simulink model "carmen_controller_HOST_prev"  (R2013b)
settings: Solver=FixedStepDiscrete  StartTime=0.0  StopTime=inf  FixedStep=0.01  RelTol=1e-3
PreLoadFcn:
  | load('motor_rule.mat');
values from neighbouring files (symbols this model uses):
  amplitud = 27000    [setup.m]
  frec = 0.1    [setup.m]
libraries: simulink x2
settings Model: Creator=Sr Antonio  LastModifiedBy=Cristina
settings DataIOCC: SignalLoggingSaveFormat=ModelDataLogs
settings OptimizationCC: ExpressionDepthLimit=2147483647
settings DebuggingCC: FcnCallInpInsideContextMsg=EnableAllAsWarning  StateNameClashWarn=warning
settings GRTTargetCC: CombineOutputUpdateFcns=off  GRTInterface=on

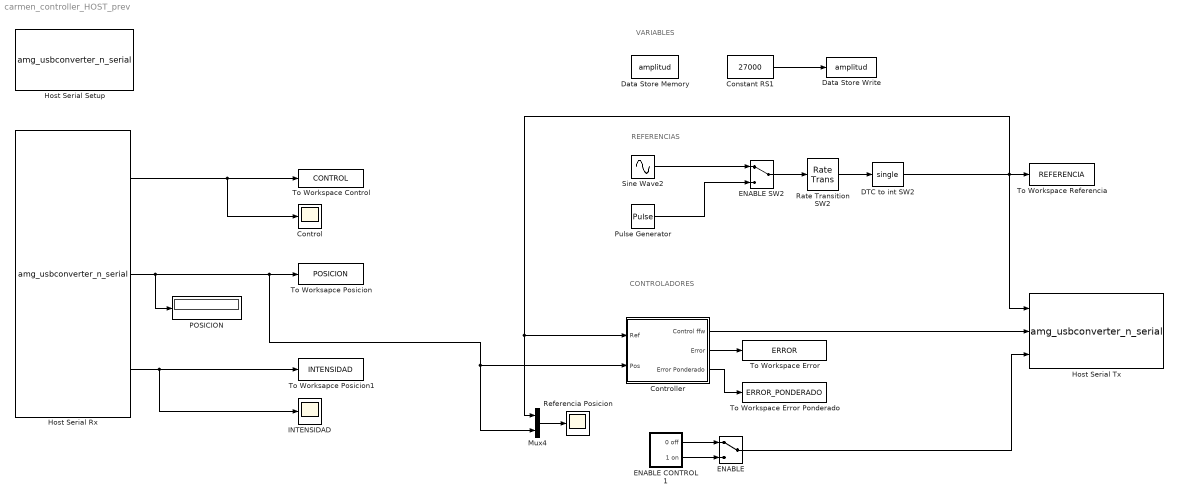
== system carmen_controller_HOST_prev ==
  note: REFERENCIAS
  note: CONTROLADORES
  note: VARIABLES
  Constant RS1 : Constant  Value=27000  OutDataTypeStr=single  SampleTime=0.01
  Control : Scope
      settings: TimeRange=10  YMin=0  YMax=37.5
  Controller : Subsystem
  DTC to int SW2 : DataTypeConversion  OutDataTypeStr=single
  Data Store Memory : DataStoreMemory  DataStoreName=amplitud  ReadBeforeWriteMsg=warning  WriteAfterWriteMsg=warning  WriteAfterReadMsg=warning
  Data Store Write : DataStoreWrite  DataStoreName=amplitud
  ENABLE : ManualSwitch
  ENABLE SW2 : ManualSwitch
  ENABLE CONTROL 1 : Subsystem
  Host Serial Rx : S-Function  Priority=1  FunctionName=amg_usbconverter_n_serial  Parameters=configuration,port,transfer,baudrate,stopbit,inputtype,outputtype,binheaderarray,binterminatorarray,asciiheader,asciiterminator,bindatalength,packetmode,timeout,sampletime,initialvalues,blockid  EnableBusSupport=off  mask(amg_usbconverter_n_serial){configuration=Rx, port=COM3, baudrate=115200, databits=8, parity=None, stopbit=1, flowcontrol=None, advanceoptions=off, rxbuffersize=2048, txbuffersize=2048, transfer=Blocking, enableinitial=off, initialvalues=[], timeout=2, packetmode=Binary, binheader='0E 0E', binterminator='0A 0A', porttype_double=0, porttype_single=3, porttype_int8=0, porttype_uint8=0, porttype_int16=0, porttype_uint16=0, porttype_int32=0, porttype_uint32=0, asciiformat='%d,%f', rx_asciiterminator=LF (0x0A - "\n"), tx_asciiterminator=LF (0x0A - "\n"), inputtype=[0], outputtype=[3  1 1 1], binheaderarray=[2 14  14], binterminatorarray=[2 10  10], bindatalength=12, asciiheader=['%d,%f' uint8(10)], asciiterminator=[1 10], sampletime=0.01, sampletimestr=, blockid=HostSerialRx}
      mask prompts: baudrate "Baud rate (bps)"; databits "Data bits"; stopbit "Stop bit"; flowcontrol "Hardware flow control"; advanceoptions "Advance options"; rxbuffersize "Rx buffer size (bytes)"; txbuffersize "Tx buffer size (bytes)"; enableinitial "Enable initial value  (Closed loop HIL test)"; initialvalues "Initial values"; timeout "Wait time-out (Seconds)"; packetmode "Packet mode"; binheader "Binary header (example: '7E 7E')"; binterminator "Binary terminator (example: '03 03')"; porttype_double "Number of data port, type DOUBLE"; porttype_single "Number of data port, type SINGLE"; porttype_int8 "Number of data port, type INT8"; porttype_uint8 "Number of data port, type UINT8"; porttype_int16 "Number of data port, type INT16"; porttype_uint16 "Number of data port, type UINT16"; porttype_int32 "Number of data port, type INT32"; porttype_uint32 "Number of data port, type UINT32"; asciiformat "Ascii format"; rx_asciiterminator "End of packet"; tx_asciiterminator "End of packet"; inputtype "Input data type"; outputtype "Output data type"; binheaderarray "Binary header"; binterminatorarray "Binary terminator"; bindatalength "Binary data length"; asciiheader "Ascii header (printf format)"; asciiterminator "Ascii terminator"; sampletime "Sample time (sec)"; sampletimestr "Compiled sample time (sec) in string"
      mask help:
      | Enable initial value (Closed loop HIL test):
      |  - Checked: The block will return a initial value (constant) at first time step.
      |  - Unchecked: Normal operation, the block waiting for matched packet data before return value.
      mask init:
      | amg_usbconverter_n_serial_callback('init');
      mask Help: web(fullfile(waijungdocroot,'amg_usbconverter_n_uart.htm'), '-browser')
      mask TypeOptions configuration: Setup | Tx | Rx
      mask Callback configuration: amg_usbconverter_n_serial_callback('configuration');
      mask TypeOptions port: COM1 | COM3
      mask Callback port: amg_usbconverter_n_serial_callback('port');
      mask Callback baudrate: amg_usbconverter_n_serial_callback('baudrate');
      mask TypeOptions databits: 8
      mask TypeOptions parity: None
      mask TypeOptions stopbit: 1 | 1.5 | 2
      mask TypeOptions flowcontrol: None | RTS | CTS | RTS/CTS
      mask Callback flowcontrol: amg_usbconverter_n_serial_callback('flowcontrol');
      mask Callback advanceoptions: amg_usbconverter_n_serial_callback('advanceoptions');
      mask TypeOptions rxbuffersize: 16 | 32 | 64 | 128 | 256 | 512 | 1024 | 2048
      mask TypeOptions txbuffersize: 16 | 32 | 64 | 128 | 256 | 512 | 1024 | 2048
      mask TypeOptions transfer: Blocking | Non-Blocking
      mask Callback transfer: amg_usbconverter_n_serial_callback('transfer');
      mask Callback enableinitial: amg_usbconverter_n_serial_callback('enableinitial');
      mask Callback initialvalues: amg_usbconverter_n_serial_callback('initialvalues');
      mask TypeOptions packetmode: Ascii | Binary
      mask Callback packetmode: amg_usbconverter_n_serial_callback('packetmode');
      mask Callback binheader: amg_usbconverter_n_serial_callback('binheader');
      mask Callback binterminator: amg_usbconverter_n_serial_callback('binterminator');
      mask Callback porttype_double: amg_usbconverter_n_serial_callback('porttype');
      mask Callback porttype_single: amg_usbconverter_n_serial_callback('porttype');
      mask Callback porttype_int8: amg_usbconverter_n_serial_callback('porttype');
      mask Callback porttype_uint8: amg_usbconverter_n_serial_callback('porttype');
      mask Callback porttype_int16: amg_usbconverter_n_serial_callback('porttype');
      mask Callback porttype_uint16: amg_usbconverter_n_serial_callback('porttype');
      mask Callback porttype_int32: amg_usbconverter_n_serial_callback('porttype');
      mask Callback porttype_uint32: amg_usbconverter_n_serial_callback('porttype');
      mask Callback asciiformat: amg_usbconverter_n_serial_callback('asciiformat');
      mask TypeOptions rx_asciiterminator: CR (0x0D - "\r") | LF (0x0A - "\n") | CRLF (0x0D 0x0A - "\r\n")
      mask Callback rx_asciiterminator: amg_usbconverter_n_serial_callback('rx_asciiterminator');
      mask TypeOptions tx_asciiterminator: CR (0x0D - "\r") | LF (0x0A - "\n") | CRLF (0x0D 0x0A - "\r\n") | None
      mask Callback tx_asciiterminator: amg_usbconverter_n_serial_callback('tx_asciiterminator');
      mask Callback sampletime: amg_usbconverter_n_serial_callback('sampletime');
      mask Callback sampletimestr: amg_usbconverter_n_serial_callback('sampletimestr');
      mask Callback blockid: amg_usbconverter_n_serial_callback('blockid');
      mask Display: text(0.05, 0.5, 'Port: COM3\nPacket: Binary\nTransfer: Blocking\nTs (sec): 0','ver','middle','hor','left');port_label('output', 1,'single');port_label('output', 2,'single');port_label('output', 3,'single');
  Host Serial Setup : S-Function  Priority=1  FunctionName=amg_usbconverter_n_serial  Parameters=configuration,port,transfer,baudrate,stopbit,inputtype,outputtype,binheaderarray,binterminatorarray,asciiheader,asciiterminator,bindatalength,packetmode,timeout,sampletime,sampletimestr,blockid  EnableBusSupport=off  mask(amg_usbconverter_n_serial){configuration=Setup, port=COM3, baudrate=10000000, databits=8, parity=None, stopbit=1, flowcontrol=None, advanceoptions=on, rxbuffersize=2048, txbuffersize=2048, transfer=Blocking, timeout=5, packetmode=Binary, binheader='7E 7E', binterminator='03 03', porttype_double=1, porttype_single=0, porttype_int8=1, porttype_uint8=0, porttype_int16=0, porttype_uint16=0, porttype_int32=0, porttype_uint32=0, asciiformat='%d,%f', rx_asciiterminator=CRLF (0x0D 0x0A - "\r\n"), tx_asciiterminator=CR (0x0D - "\r"), inputtype=[0], outputtype=[0], binheaderarray=[2 126  126], binterminatorarray=[2 3  3], bindatalength=0, asciiheader='', asciiterminator=[0], sampletime=inf, sampletimestr=, blockid=HostSerialSetup}
      mask prompts: baudrate "Baud rate (bps)"; databits "Data bits"; stopbit "Stop bit"; flowcontrol "Hardware flow control"; advanceoptions "Advance options"; rxbuffersize "Rx buffer size (bytes)"; txbuffersize "Tx buffer size (bytes)"; timeout "Wait time-out (Seconds)"; packetmode "Packet mode"; binheader "Binary header (example: '7E 7E')"; binterminator "Binary terminator (example: '03 03')"; porttype_double "Number of data port, type DOUBLE"; porttype_single "Number of data port, type SINGLE"; porttype_int8 "Number of data port, type INT8"; porttype_uint8 "Number of data port, type UINT8"; porttype_int16 "Number of data port, type INT16"; porttype_uint16 "Number of data port, type UINT16"; porttype_int32 "Number of data port, type INT32"; porttype_uint32 "Number of data port, type UINT32"; asciiformat "Ascii format"; rx_asciiterminator "End of packet"; tx_asciiterminator "End of packet"; inputtype "Input data type"; outputtype "Output data type"; binheaderarray "Binary header"; binterminatorarray "Binary terminator"; bindatalength "Binary data length"; asciiheader "Ascii header (printf format)"; asciiterminator "Ascii terminator"; sampletime "Sample time (sec)"; sampletimestr "Compiled sample time (sec) in string"
      mask init:
      | amg_usbconverter_n_serial_callback('init');
      mask Help: web(fullfile(waijungdocroot,'amg_usbconverter_n_uart.htm'), '-browser')
      mask TypeOptions configuration: Setup | Tx | Rx
      mask Callback configuration: amg_usbconverter_n_serial_callback('configuration');
      mask TypeOptions port: COM1 | COM3
      mask Callback port: amg_usbconverter_n_serial_callback('port');
      mask Callback baudrate: amg_usbconverter_n_serial_callback('baudrate');
      mask TypeOptions databits: 8
      mask TypeOptions parity: None
      mask TypeOptions stopbit: 1 | 1.5 | 2
      mask TypeOptions flowcontrol: None | RTS | CTS | RTS/CTS
      mask Callback flowcontrol: amg_usbconverter_n_serial_callback('flowcontrol');
      mask Callback advanceoptions: amg_usbconverter_n_serial_callback('advanceoptions');
      mask TypeOptions rxbuffersize: 16 | 32 | 64 | 128 | 256 | 512 | 1024 | 2048
      mask TypeOptions txbuffersize: 16 | 32 | 64 | 128 | 256 | 512 | 1024 | 2048
      mask TypeOptions transfer: Blocking | Non-Blocking
      mask Callback transfer: amg_usbconverter_n_serial_callback('transfer');
      mask TypeOptions packetmode: Ascii | Binary
      mask Callback packetmode: amg_usbconverter_n_serial_callback('packetmode');
      mask Callback binheader: amg_usbconverter_n_serial_callback('binheader');
      mask Callback binterminator: amg_usbconverter_n_serial_callback('binterminator');
      mask Callback porttype_double: amg_usbconverter_n_serial_callback('porttype');
      mask Callback porttype_single: amg_usbconverter_n_serial_callback('porttype');
      mask Callback porttype_int8: amg_usbconverter_n_serial_callback('porttype');
      mask Callback porttype_uint8: amg_usbconverter_n_serial_callback('porttype');
      mask Callback porttype_int16: amg_usbconverter_n_serial_callback('porttype');
      mask Callback porttype_uint16: amg_usbconverter_n_serial_callback('porttype');
      mask Callback porttype_int32: amg_usbconverter_n_serial_callback('porttype');
      mask Callback porttype_uint32: amg_usbconverter_n_serial_callback('porttype');
      mask Callback asciiformat: amg_usbconverter_n_serial_callback('asciiformat');
      mask TypeOptions rx_asciiterminator: CR (0x0D - "\r") | LF (0x0A - "\n") | CRLF (0x0D 0x0A - "\r\n")
      mask Callback rx_asciiterminator: amg_usbconverter_n_serial_callback('rx_asciiterminator');
      mask TypeOptions tx_asciiterminator: CR (0x0D - "\r") | LF (0x0A - "\n") | CRLF (0x0D 0x0A - "\r\n") | None
      mask Callback tx_asciiterminator: amg_usbconverter_n_serial_callback('tx_asciiterminator');
      mask Callback sampletime: amg_usbconverter_n_serial_callback('sampletime');
      mask Callback sampletimestr: amg_usbconverter_n_serial_callback('sampletimestr');
      mask Callback blockid: amg_usbconverter_n_serial_callback('blockid');
      mask Display: text(0.5, 0.5, 'Port: COM3\nBaud (Bps): 10000000\nFrame: 8-None-1','ver','middle','hor','center');
  Host Serial Tx : S-Function  Priority=1  FunctionName=amg_usbconverter_n_serial  Parameters=configuration,port,transfer,baudrate,stopbit,inputtype,outputtype,binheaderarray,binterminatorarray,asciiheader,asciiterminator,bindatalength,packetmode,timeout,sampletime,sampletimestr,blockid  EnableBusSupport=off  mask(amg_usbconverter_n_serial){configuration=Tx, port=COM3, baudrate=115200, databits=8, parity=None, stopbit=1, flowcontrol=None, advanceoptions=off, rxbuffersize=2048, txbuffersize=2048, transfer=Blocking, timeout=2, packetmode=Binary, binheader='0E 0E', binterminator='0A 0A', porttype_double=0, porttype_single=2, porttype_int8=0, porttype_uint8=1, porttype_int16=0, porttype_uint16=0, porttype_int32=0, porttype_uint32=0, asciiformat='%d,%f', rx_asciiterminator=CRLF (0x0D 0x0A - "\r\n"), tx_asciiterminator=LF (0x0A - "\n"), inputtype=[3  1 1 3], outputtype=[0], binheaderarray=[2 14  14], binterminatorarray=[2 10  10], bindatalength=9, asciiheader=['%d,%f' uint8(10)], asciiterminator=[1 10], sampletime=0.01, sampletimestr=, blockid=HostSerialTx}
      mask prompts: baudrate "Baud rate (bps)"; databits "Data bits"; stopbit "Stop bit"; flowcontrol "Hardware flow control"; advanceoptions "Advance options"; rxbuffersize "Rx buffer size (bytes)"; txbuffersize "Tx buffer size (bytes)"; timeout "Wait time-out (Seconds)"; packetmode "Packet mode"; binheader "Binary header (example: '7E 7E')"; binterminator "Binary terminator (example: '03 03')"; porttype_double "Number of data port, type DOUBLE"; porttype_single "Number of data port, type SINGLE"; porttype_int8 "Number of data port, type INT8"; porttype_uint8 "Number of data port, type UINT8"; porttype_int16 "Number of data port, type INT16"; porttype_uint16 "Number of data port, type UINT16"; porttype_int32 "Number of data port, type INT32"; porttype_uint32 "Number of data port, type UINT32"; asciiformat "Ascii format"; rx_asciiterminator "End of packet"; tx_asciiterminator "End of packet"; inputtype "Input data type"; outputtype "Output data type"; binheaderarray "Binary header"; binterminatorarray "Binary terminator"; bindatalength "Binary data length"; asciiheader "Ascii header (printf format)"; asciiterminator "Ascii terminator"; sampletime "Sample time (sec)"; sampletimestr "Compiled sample time (sec) in string"
      mask init:
      | amg_usbconverter_n_serial_callback('init');
      mask Help: web(fullfile(waijungdocroot,'amg_usbconverter_n_uart.htm'), '-browser')
      mask TypeOptions configuration: Setup | Tx | Rx
      mask Callback configuration: amg_usbconverter_n_serial_callback('configuration');
      mask TypeOptions port: COM1 | COM3
      mask Callback port: amg_usbconverter_n_serial_callback('port');
      mask Callback baudrate: amg_usbconverter_n_serial_callback('baudrate');
      mask TypeOptions databits: 8
      mask TypeOptions parity: None
      mask TypeOptions stopbit: 1 | 1.5 | 2
      mask TypeOptions flowcontrol: None | RTS | CTS | RTS/CTS
      mask Callback flowcontrol: amg_usbconverter_n_serial_callback('flowcontrol');
      mask Callback advanceoptions: amg_usbconverter_n_serial_callback('advanceoptions');
      mask TypeOptions rxbuffersize: 16 | 32 | 64 | 128 | 256 | 512 | 1024 | 2048
      mask TypeOptions txbuffersize: 16 | 32 | 64 | 128 | 256 | 512 | 1024 | 2048
      mask TypeOptions transfer: Blocking | Non-Blocking
      mask Callback transfer: amg_usbconverter_n_serial_callback('transfer');
      mask TypeOptions packetmode: Ascii | Binary
      mask Callback packetmode: amg_usbconverter_n_serial_callback('packetmode');
      mask Callback binheader: amg_usbconverter_n_serial_callback('binheader');
      mask Callback binterminator: amg_usbconverter_n_serial_callback('binterminator');
      mask Callback porttype_double: amg_usbconverter_n_serial_callback('porttype');
      mask Callback porttype_single: amg_usbconverter_n_serial_callback('porttype');
      mask Callback porttype_int8: amg_usbconverter_n_serial_callback('porttype');
      mask Callback porttype_uint8: amg_usbconverter_n_serial_callback('porttype');
      mask Callback porttype_int16: amg_usbconverter_n_serial_callback('porttype');
      mask Callback porttype_uint16: amg_usbconverter_n_serial_callback('porttype');
      mask Callback porttype_int32: amg_usbconverter_n_serial_callback('porttype');
      mask Callback porttype_uint32: amg_usbconverter_n_serial_callback('porttype');
      mask Callback asciiformat: amg_usbconverter_n_serial_callback('asciiformat');
      mask TypeOptions rx_asciiterminator: CR (0x0D - "\r") | LF (0x0A - "\n") | CRLF (0x0D 0x0A - "\r\n")
      mask Callback rx_asciiterminator: amg_usbconverter_n_serial_callback('rx_asciiterminator');
      mask TypeOptions tx_asciiterminator: CR (0x0D - "\r") | LF (0x0A - "\n") | CRLF (0x0D 0x0A - "\r\n") | None
      mask Callback tx_asciiterminator: amg_usbconverter_n_serial_callback('tx_asciiterminator');
      mask Callback sampletime: amg_usbconverter_n_serial_callback('sampletime');
      mask Callback sampletimestr: amg_usbconverter_n_serial_callback('sampletimestr');
      mask Callback blockid: amg_usbconverter_n_serial_callback('blockid');
      mask Display: text(0.95, 0.5, 'Port: COM3\nPacket: Binary\nTransfer: Blocking\nTs (sec): 0','ver','middle','hor','right');port_label('input', 1,'single');port_label('input', 2,'single');port_label('input', 3,'uint8');
  INTENSIDAD : Scope
      settings: TimeRange=10  YMin=-100  YMax=2000  SaveName=ScopeData5
  Mux4 : Mux  Inputs=2
  POSICION : Display
  Pulse Generator : DiscretePulseGenerator  PulseType=Time based  Amplitude=54000  Period=60  PulseWidth=20
  Rate Transition SW2 : RateTransition  OutPortSampleTime=0.01
  Referencia Posicion : Scope
      settings: TimeRange=100  YMin=0  YMax=20000  SaveName=ScopeData7  MaxDataPoints=50000
  Sine Wave2 : Sin  Amplitude=amplitud  Bias=amplitud  Frequency=frec  Phase=-pi/2  SampleTime=0
  To Worksapce Posicion : ToWorkspace  VariableName=POSICION  SampleTime=-1  SaveFormat=Structure With Time
  To Worksapce Posicion1 : ToWorkspace  VariableName=INTENSIDAD  SampleTime=-1  SaveFormat=Structure With Time
  To Workspace Control : ToWorkspace  VariableName=CONTROL  SampleTime=-1  SaveFormat=Structure With Time
  To Workspace Error : ToWorkspace  VariableName=ERROR  SampleTime=-1  SaveFormat=Structure
  To Workspace Error Ponderado : ToWorkspace  VariableName=ERROR_PONDERADO  SampleTime=-1  SaveFormat=Structure
  To Workspace Referencia : ToWorkspace  VariableName=REFERENCIA  SampleTime=-1  SaveFormat=Structure With Time
  wires:
  ENABLE CONTROL 1/1(0 off) -> ENABLE/1
  ENABLE CONTROL 1/2(1 on) -> ENABLE/2
  Rate Transition SW2/1 -> DTC to int SW2/1
  DTC to int SW2/1 -> Host Serial Tx/1, Controller/1(Ref), Mux4/1, To Workspace Referencia/1
  ENABLE SW2/1 -> Rate Transition SW2/1
  Controller/1(Control ffw) -> Host Serial Tx/2
  Mux4/1 -> Referencia Posicion/1
  Host Serial Rx/3 -> INTENSIDAD/1, To Worksapce Posicion1/1
  Constant RS1/1 -> Data Store Write/1
  Sine Wave2/1 -> ENABLE SW2/1
  Pulse Generator/1 -> ENABLE SW2/2
  ENABLE/1 -> Host Serial Tx/3
  Host Serial Rx/1 -> Control/1, To Workspace Control/1
  Host Serial Rx/2 -> Controller/2(Pos), Mux4/2, To Worksapce Posicion/1, POSICION/1
  Controller/2(Error) -> To Workspace Error/1
  Controller/3(Error Ponderado) -> To Workspace Error Ponderado/1

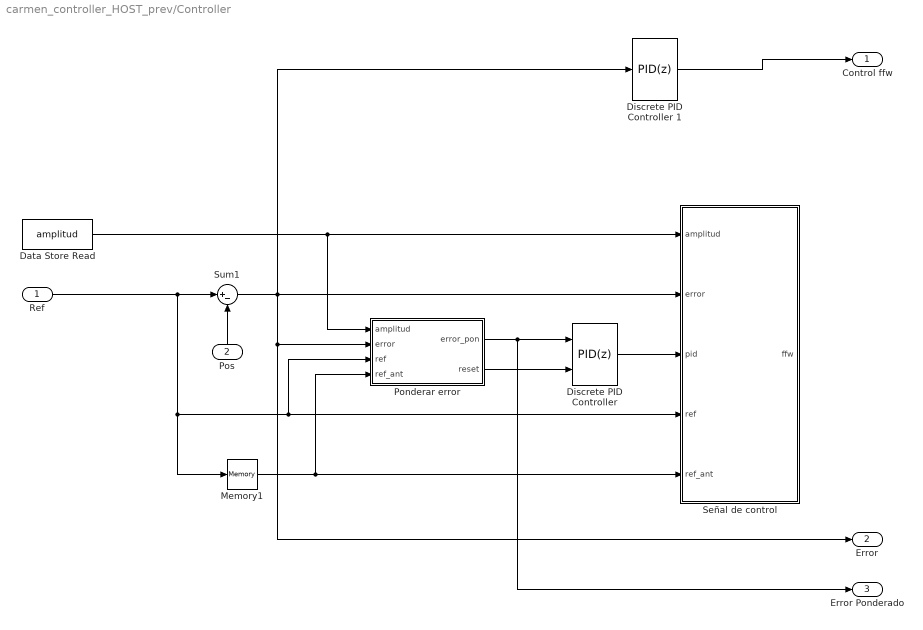
== system carmen_controller_HOST_prev/Controller ==
  Ref : Inport
  Pos : Inport  Port=2
  Data Store Read : DataStoreRead  DataStoreName=amplitud
  "Discrete PID Controller " : simulink/Continuous/PID Controller  Controller=PID  TimeDomain=Discrete-time  SampleTime=0.01  IntegratorMethod=Forward Euler  FilterMethod=Forward Euler  Form=Parallel  P=0.24  I=0  D=0.01  N=100  InitialConditionSource=internal  InitialConditionForIntegrator=0  InitialConditionForFilter=0  ExternalReset=rising  LimitOutput=off  UpperSaturationLimit=inf  LowerSaturationLimit=-50  LinearizeAsGain=off  AntiWindupMode=none  Kb=1  TrackingMode=off  Kt=1  PParamMin=[]  PParamMax=[]  IParamMin=[]  IParamMax=[]  DParamMin=[]  DParamMax=[]  NParamMin=[]  NParamMax=[]  KbParamMin=[]  KbParamMax=[]  KtParamMin=[]  KtParamMax=[]  POutMin=[]  POutMax=[]  IOutMin=[]  IOutMax=[]  DOutMin=[]  DOutMax=[]  NOutMin=[]  NOutMax=[]  KbOutMin=[]  KbOutMax=[]  KtOutMin=[]  KtOutMax=[]  IntegratorOutMin=[]  IntegratorOutMax=[]  FilterOutMin=[]  FilterOutMax=[]  SumOutMin=[]  SumOutMax=[]  SumI1OutMin=[]  SumI1OutMax=[]  SumI2OutMin=[]  SumI2OutMax=[]  SumI3OutMin=[]  SumI3OutMax=[]  SumDOutMin=[]  SumDOutMax=[]  SaturationOutMin=[]  SaturationOutMax=[]  IntegratorContinuousStateAttributes=''  IntegratorStateMustResolveToSignalObject=off  IntegratorRTWStateStorageClass=Auto  FilterContinuousStateAttributes=''  FilterStateMustResolveToSignalObject=off  FilterRTWStateStorageClass=Auto
  Discrete PID Controller 1 : simulink/Continuous/PID Controller  Controller=PID  TimeDomain=Discrete-time  SampleTime=0.01  IntegratorMethod=Forward Euler  FilterMethod=Forward Euler  Form=Parallel  P=0.024  I=0  D=0.001  N=100  InitialConditionSource=internal  InitialConditionForIntegrator=0  InitialConditionForFilter=0  ExternalReset=none  LimitOutput=off  UpperSaturationLimit=inf  LowerSaturationLimit=-50  LinearizeAsGain=off  AntiWindupMode=none  Kb=1  TrackingMode=off  Kt=1  PParamMin=[]  PParamMax=[]  IParamMin=[]  IParamMax=[]  DParamMin=[]  DParamMax=[]  NParamMin=[]  NParamMax=[]  KbParamMin=[]  KbParamMax=[]  KtParamMin=[]  KtParamMax=[]  POutMin=[]  POutMax=[]  IOutMin=[]  IOutMax=[]  DOutMin=[]  DOutMax=[]  NOutMin=[]  NOutMax=[]  KbOutMin=[]  KbOutMax=[]  KtOutMin=[]  KtOutMax=[]  IntegratorOutMin=[]  IntegratorOutMax=[]  FilterOutMin=[]  FilterOutMax=[]  SumOutMin=[]  SumOutMax=[]  SumI1OutMin=[]  SumI1OutMax=[]  SumI2OutMin=[]  SumI2OutMax=[]  SumI3OutMin=[]  SumI3OutMax=[]  SumDOutMin=[]  SumDOutMax=[]  SaturationOutMin=[]  SaturationOutMax=[]  IntegratorContinuousStateAttributes=''  IntegratorStateMustResolveToSignalObject=off  IntegratorRTWStateStorageClass=Auto  FilterContinuousStateAttributes=''  FilterStateMustResolveToSignalObject=off  FilterRTWStateStorageClass=Auto
  Memory1 : Memory  InheritSampleTime=on
  Ponderar error : MATLAB Function  TreatAsAtomicUnit=on
  Señal de control : MATLAB Function  TreatAsAtomicUnit=on
  Sum1 : Sum  Inputs=|+-
  Control ffw : Outport
  Error : Outport  Port=2
  Error Ponderado : Outport  Port=3
  wires:
  Pos/1 -> Sum1/2
  Ref/1 -> Ponderar error/3(ref), Señal de control/4(ref), Memory1/1, Sum1/1
  Sum1/1 -> Error/1, Ponderar error/2(error), Discrete PID Controller 1/1, Señal de control/2(error)
  Ponderar error/1(error_pon) -> Error Ponderado/1, "Discrete PID Controller "/1
  "Discrete PID Controller "/1 -> Señal de control/3(pid)
  Memory1/1 -> Ponderar error/4(ref_ant), Señal de control/5(ref_ant)
  Data Store Read/1 -> Señal de control/1(amplitud), Ponderar error/1(amplitud)
  Ponderar error/2(reset) -> "Discrete PID Controller "/2
  Discrete PID Controller 1/1 -> Control ffw/1

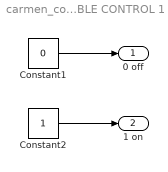
== system carmen_controller_HOST_prev/ENABLE CONTROL 1 ==
  Constant1 : Constant  Value=0  OutDataTypeStr=uint8  SampleTime=0.01
  Constant2 : Constant  OutDataTypeStr=uint8
  0 off : Outport
  1 on : Outport  Port=2
  wires:
  Constant2/1 -> 1 on/1
  Constant1/1 -> 0 off/1

== matlab function carmen_controller_HOST_prev/Controller/Señal de control ==
  data: amplitud input; error input; ffw output; pid input; ref input; ref_ant input
function ffw = fcn(amplitud, error, pid, ref, ref_ant)
%     if pid > 40
%         pid = 40;
%     end
    
    % Primer caso: maxima amplitud
    if (ref > amplitud*2*0.98) && (ref_ant < ref)
        if (error < -50)
           ffw = single(0);
       else
           ffw = single(pid*0.75);
        end

    % Segundo caso: referencia descendente
    elseif (ref_ant > ref)
       if (error < -500)
           ffw = single(0);
       else
           ffw = single(pid);
       end

    % Tercer caso: referencia ascendente
    else
        if (error < -500)
           ffw = single(max(0, 2-(0.002*abs(error))));
        else
           ffw = single(pid);
        end
    end
end

== matlab function carmen_controller_HOST_prev/Controller/Ponderar error ==
  data: amplitud input; error input; ref input; error_pon output; ref_ant input; reset output
function [error_pon, reset] = fcn(amplitud, error, ref, ref_ant)
    if (error < -1000) %|| (ref >= -0.05 && ref <= 0.05)
       reset = 1;
    else
       reset = 0;
    end

    % Segundo caso: referencia descendente
    if (error < -500)
        error_pon = error*0.01;
    else
       error_pon = error;
    
    end
end
